simulink model "data_logging_system"  (R2018a)
settings: Solver=VariableStepAuto  StartTime=0.0  StopTime=10.0  RelTol=1e-3
settings Model: Creator=Jarvis  LastModifiedBy=Jarvis

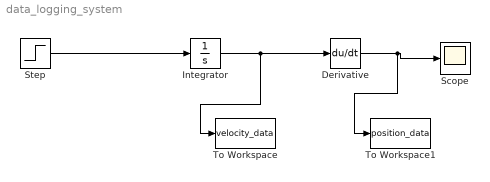
== system data_logging_system ==
  Derivative : Derivative
  Integrator : Integrator
  Scope : Scope
  Step : Step  SampleTime=0
  To Workspace : ToWorkspace  VariableName=velocity_data  SaveFormat=Timeseries  SampleTime=-1
  To Workspace1 : ToWorkspace  VariableName=position_data  SaveFormat=Timeseries  SampleTime=-1
  wires:
  Step/1 -> Integrator/1
  Derivative/1 -> To Workspace1/1, Scope/1
  Integrator/1 -> To Workspace/1, Derivative/1
